simulink model "SandboxInputPorcessing"  (R2020a)
settings: Solver=FixedStepDiscrete  StartTime=0.0  StopTime=inf  FixedStep=0.02  RelTol=1e-3
values from neighbouring files (symbols this model uses):
  ToDelete = 121.5515625    [Parameters.m]
settings Model: Creator=marqu  LastModifiedBy=marqu

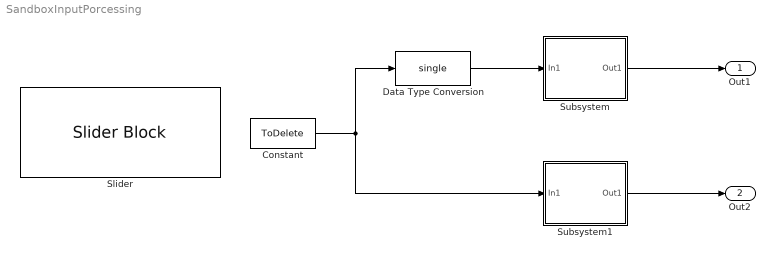
== system SandboxInputPorcessing ==
  Constant : Constant  Value=ToDelete  OutDataTypeStr=uint8
  Data Type Conversion : DataTypeConversion  OutDataTypeStr=single
  Slider : SliderBlock  ScaleMin=51  ScaleMax=204
  Subsystem : Subsystem
  Subsystem1 : Subsystem
  Out1 : Outport
  Out2 : Outport  Port=2
  wires:
  Subsystem/1(Out1) -> Out1/1
  Data Type Conversion/1 -> Subsystem/1(In1)
  Subsystem1/1(Out1) -> Out2/1
  Constant/1 -> Subsystem1/1(In1), Data Type Conversion/1

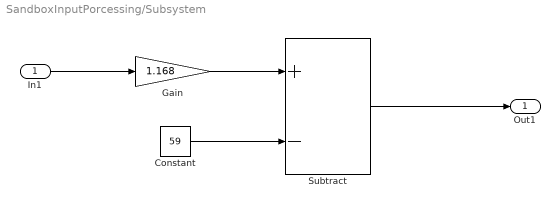
== system SandboxInputPorcessing/Subsystem ==
  In1 : Inport
  Constant : Constant  Value=59  OutDataTypeStr=uint8
  Gain : Gain  Gain=1.168
  Subtract : Sum  Inputs=+-
  Out1 : Outport
  wires:
  Constant/1 -> Subtract/2
  Gain/1 -> Subtract/1
  Subtract/1 -> Out1/1
  In1/1 -> Gain/1

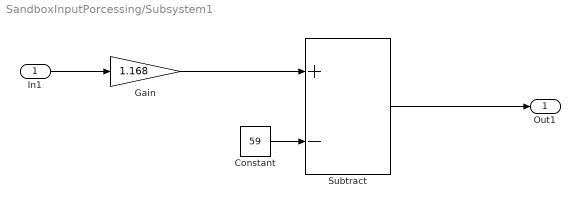
== system SandboxInputPorcessing/Subsystem1 ==
  In1 : Inport
  Constant : Constant  Value=59  OutDataTypeStr=uint8
  Gain : Gain  Gain=1.168  OutDataTypeStr=single
  Subtract : Sum  Inputs=+-  OutDataTypeStr=uint8
  Out1 : Outport
  wires:
  Constant/1 -> Subtract/2
  Gain/1 -> Subtract/1
  Subtract/1 -> Out1/1
  In1/1 -> Gain/1
